simulink model "LQG_AWBT"  (Simulink 7.1)
settings: Solver=ode5  StartTime=0.0  StopTime=0.5  FixedStep=1e-4  RelTol=1e-3
values from neighbouring files (symbols this model uses):
  Ak = [-672.634870495 -2626.58972998 -46.1193303275 25.5793500122 108.891317034 -102.718752792 -245.794654799 -577.315326704 39.8827087547 153.58157137 60.36854216 -207.81122515 ... (144 elements, 12x12)]    [controller_reduced.mat]    (also in main_matlab.m = rlqg.A)
  Bk = [0.204306341627 1.11161335273 -0.324978673641 2.85402340631 -4.5813117605 2.97328839236 -0.174709893359 1.31662160979 2.94898293865 13.5567055967 -0.791381118401 0.0552385579013]    [controller_reduced.mat]    (also in main_matlab.m = rlqg.B)
  Ck = [534.788956442 909.016401092 107.069958755 -410.092366717 -1097.26369634 478.53061829 -894.210554118 460.341899649 -450.064931583 371.993181033 532.787728171 55.8162878584 ... (24 elements, 2x12)]    [controller_reduced.mat]    (also in main_matlab.m = rlqg.C)
  Dk = [0 0]    [controller_reduced.mat]    (also in main_matlab.m = rlqg.D)
  Lambda = X/M    [main_matlab.m]
  nk = sqrt(numel(Ak))    [main_matlab.m]
  nu = numel(Bpu)/np    [main_matlab.m]
undefined symbols (not defined in the file or in its folder): Af, Bf, Cf, Hf
libraries: cstblocks x1
settings Model: Creator=p4wp4w  LastModifiedBy=Ablah
settings OptimizationCC: ExpressionDepthLimit=128  InitFltsAndDblsToZero=off
settings DebuggingCC: SolverPrmCheckMsg=none  FcnCallInpInsideContextMsg=Enable All  StateNameClashWarn=none  StrictBusMsg=ErrorLevel1
settings CodeAppCC: CustomSymbolStrType=$N$R$M_T
settings GRTTargetCC: TargetFunctionLibrary=C89/C90 (ANSI)  CPPClassGenCompliant=off

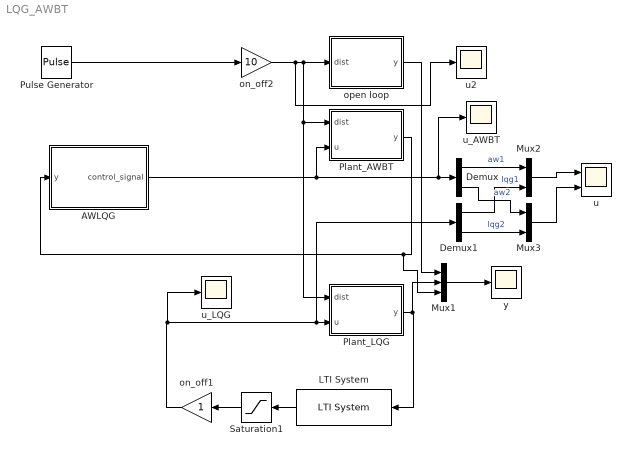
== system LQG_AWBT ==
  AWLQG : Subsystem
  Demux : Demux  Outputs=2
  Demux1 : Demux  Outputs=2
  LTI System : cstblocks/LTI System  Orientation=left  sys=rlqg  IC=[]
  Mux1 : Mux  Inputs=3
  Mux2 : Mux  Inputs=2
  Mux3 : Mux  Inputs=2
  Plant_AWBT : Subsystem
  Plant_LQG : Subsystem
  Pulse Generator : DiscretePulseGenerator  PulseType=Time based  Period=0.5  PulseWidth=10
  Saturation1 : Saturate  Orientation=left  UpperLimit=2  LowerLimit=-2
  on_off1 : Gain  Orientation=left
  on_off2 : Gain  Gain=10
  open loop : Subsystem
  u : Scope  NumInputPorts=2
      settings: YMin=-0.8~-5  YMax=0.7~5  SaveName=ScopeData3
  u2 : Scope
      settings: YMin=-0.8  YMax=0.7  SaveName=ScopeData6
  u_AWBT : Scope
      settings: YMin=-1  YMax=1
  u_LQG : Scope
      settings: SaveName=ScopeData2
  y : Scope
      settings: YMin=-15  YMax=15
  wires:
  LTI System/1 -> Saturation1/1
  Saturation1/1 -> on_off1/1
  Mux1/1 -> y/1
  open loop/1(y) -> Mux1/1
  on_off1/1 -> u_LQG/1, Demux1/1, Plant_LQG/2(u)
  on_off2/1 -> u2/1, open loop/1(dist), Plant_LQG/1(dist), Plant_AWBT/1(dist)
  Plant_LQG/1(y) -> Mux1/2, LTI System/1
  Plant_AWBT/1(y) -> AWLQG/1(y), Mux1/3
  Demux/1 -> Mux2/1  "aw1"
  Demux1/1 -> Mux2/2  "lqg1"
  Demux/2 -> Mux3/1  "aw2"
  Demux1/2 -> Mux3/2  "lqg2"
  Pulse Generator/1 -> on_off2/1
  Mux2/1 -> u/1
  Mux3/1 -> u/2
  AWLQG/1(control_signal) -> Plant_AWBT/2(u), u_AWBT/1, Demux/1

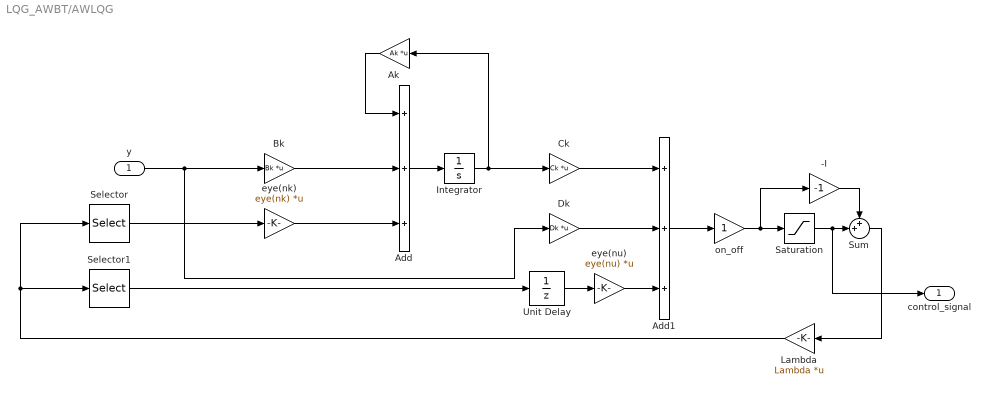
== system LQG_AWBT/AWLQG ==
  y : Inport
  -I : Gain  Gain=-1
  Add : Sum  Inputs=+++
  Add1 : Sum  Inputs=+++
  Ak : Gain  Orientation=left  Gain=Ak  Multiplication=Matrix(K*u)
  Bk : Gain  Gain=Bk  Multiplication=Matrix(K*u)
  Ck : Gain  Gain=Ck  Multiplication=Matrix(K*u)
  Dk : Gain  Gain=Dk  Multiplication=Matrix(K*u)
  Integrator : Integrator
  Lambda : Gain  Orientation=left  Gain=Lambda  Multiplication=Matrix(K*u)
  Saturation : Saturate  UpperLimit=2  LowerLimit=-2
  Selector : Selector  InputPortWidth=nk+nu  Indices=[1:nk]
  Selector1 : Selector  InputPortWidth=nk+nu  Indices=[nk+1:nk+nu]
  Sum : Sum  Inputs=++|
  Unit Delay : UnitDelay  SampleTime=-1
  eye(nk) : Gain  Gain=eye(nk)  Multiplication=Matrix(K*u)
  eye(nu) : Gain  Gain=eye(nu)  Multiplication=Matrix(K*u)
  on_off : Gain
  control_signal : Outport
  wires:
  Lambda/1 -> Selector1/1, Selector/1
  -I/1 -> Sum/1
  Sum/1 -> Lambda/1
  Add1/1 -> on_off/1
  Saturation/1 -> control_signal/1, Sum/2
  on_off/1 -> -I/1, Saturation/1
  Add/1 -> Integrator/1
  Integrator/1 -> Ak/1, Ck/1
  Ak/1 -> Add/1
  Bk/1 -> Add/2
  y/1 -> Dk/1, Bk/1
  eye(nk)/1 -> Add/3
  Selector/1 -> eye(nk)/1
  Ck/1 -> Add1/1
  Dk/1 -> Add1/2
  eye(nu)/1 -> Add1/3
  Selector1/1 -> Unit Delay/1
  Unit Delay/1 -> eye(nu)/1

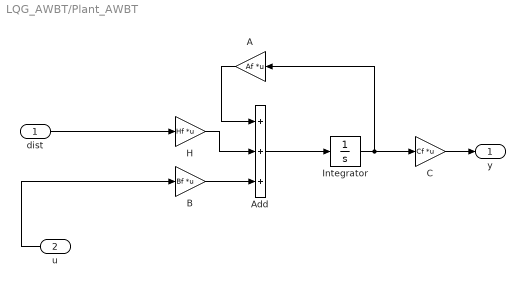
== system LQG_AWBT/Plant_AWBT ==
  dist : Inport
  u : Inport  Orientation=left  Port=2
  A : Gain  Orientation=left  Gain=Af  Multiplication=Matrix(K*u)
  Add : Sum  Inputs=+++
  B : Gain  Gain=Bf  Multiplication=Matrix(K*u)
  C : Gain  Gain=Cf  Multiplication=Matrix(K*u)
  H : Gain  Gain=Hf  Multiplication=Matrix(K*u)
  Integrator : Integrator
  y : Outport
  wires:
  Add/1 -> Integrator/1
  H/1 -> Add/2
  A/1 -> Add/1
  dist/1 -> H/1
  C/1 -> y/1
  B/1 -> Add/3
  Integrator/1 -> C/1, A/1
  u/1 -> B/1

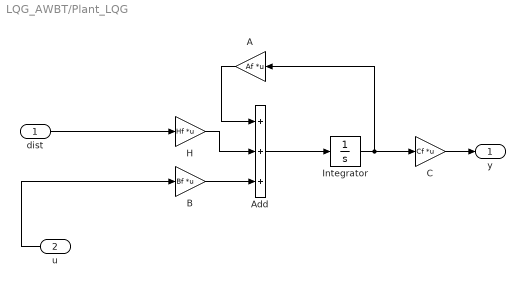
== system LQG_AWBT/Plant_LQG ==
  dist : Inport
  u : Inport  Orientation=left  Port=2
  A : Gain  Orientation=left  Gain=Af  Multiplication=Matrix(K*u)
  Add : Sum  Inputs=+++
  B : Gain  Gain=Bf  Multiplication=Matrix(K*u)
  C : Gain  Gain=Cf  Multiplication=Matrix(K*u)
  H : Gain  Gain=Hf  Multiplication=Matrix(K*u)
  Integrator : Integrator
  y : Outport
  wires:
  u/1 -> B/1
  Integrator/1 -> A/1, C/1
  B/1 -> Add/3
  C/1 -> y/1
  dist/1 -> H/1
  A/1 -> Add/1
  H/1 -> Add/2
  Add/1 -> Integrator/1

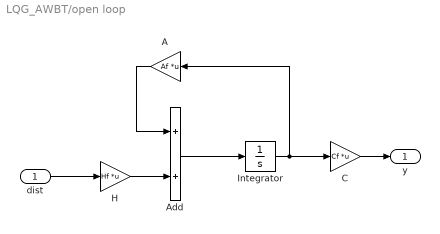
== system LQG_AWBT/open loop ==
  dist : Inport
  A : Gain  Orientation=left  Gain=Af  Multiplication=Matrix(K*u)
  Add : Sum
  C : Gain  Gain=Cf  Multiplication=Matrix(K*u)
  H : Gain  Gain=Hf  Multiplication=Matrix(K*u)
  Integrator : Integrator
  y : Outport
  wires:
  Integrator/1 -> A/1, C/1
  C/1 -> y/1
  dist/1 -> H/1
  A/1 -> Add/1
  H/1 -> Add/2
  Add/1 -> Integrator/1
